simulink model "fixed_model"  (R2024a)
settings: Solver=VariableStepAuto  StartTime=0.0  StopTime=2  RelTol=1e-3
undefined symbols (not defined in the file or in its folder): Radix, SAMPLING_FREQ, signal_1
libraries: dspstat3 x3, dspsrcs4 x1, dspxfrm3 x1, simulink x1
settings Model: SimulationMode=accelerator  Creator=Jan Rosa  LastModifiedBy=Jan Rosa
settings DebuggingCC: SignalRangeChecking=warning
settings HardwareCC: ProdBitPerPointer=32  ProdBitPerSizeT=32  ProdBitPerPtrDiffT=32  ProdLargestAtomicFloat=None  ProdIntDivRoundTo=Undefined  ProdEndianess=Unspecified  ProdWordSize=32  ProdHWDeviceType=ASIC/FPGA->ASIC/FPGA  TargetBitPerPointer=64  TargetBitPerSizeT=64  TargetBitPerPtrDiffT=64  TargetLongLongMode=on  TargetIntDivRoundTo=Zero  TargetEndianess=LittleEndian  TargetWordSize=64  TargetHWDeviceType=Custom Processor->MATLAB Host Computer  ProdEqTarget=off

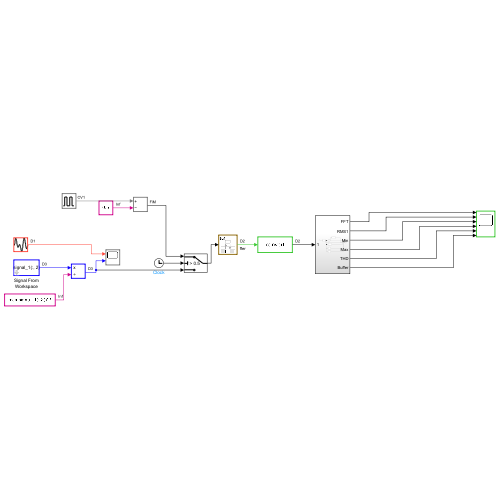
[thumbnail: Simulink's stored preview of the top-level diagram]
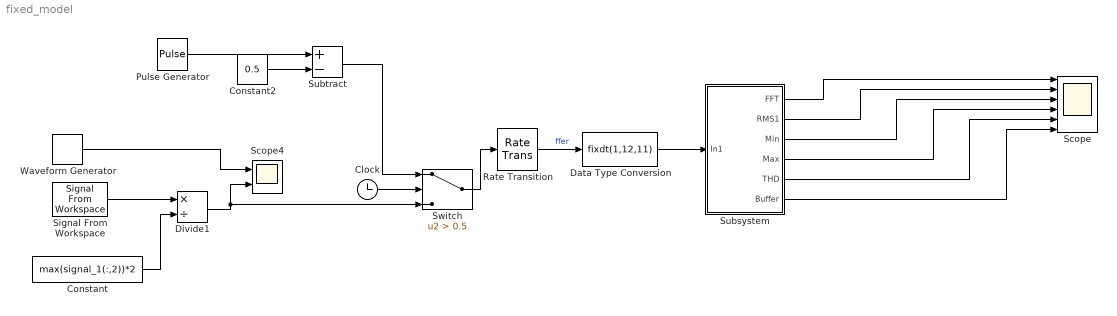
== system fixed_model ==
  Clock : Clock
  Constant : Constant  Value=max(signal_1(:,2))*2
  Constant2 : Constant  Value=0.5
  Data Type Conversion : DataTypeConversion  OutDataTypeStr=fixdt(1,12,11)  SaturateOnIntegerOverflow=off  RndMeth=Floor
  Divide1 : Product  Inputs=*/
  Pulse Generator : DiscretePulseGenerator  PulseType=Time based  Amplitude=0.999  Period=1/50  PulseWidth=50
  Rate Transition : RateTransition  Deterministic=off  OutPortSampleTime=1/SAMPLING_FREQ
  Scope : Scope  NumInputPorts=6
  Scope4 : Scope  NumInputPorts=2
  Signal From Workspace : dspsrcs4/Signal From Workspace  X=signal_1(:, 2)  Ts=signal_1(2, 1)  nsamps=1  OutputAfterFinalValue=Cyclic repetition  ignoreOrWarnInputAndFrameLengths=off  OutputFrames=off
  Subsystem : Subsystem
  Subtract : Sum  Inputs=+-
  Switch : Switch  Criteria=u2 > Threshold  Threshold=0.5  SaturateOnIntegerOverflow=off  InputSameDT=off
  Waveform Generator : simulink/Sources/Waveform Generator  OutMin=[]  OutMax=[]  OutDataTypeStr=double  SelectedSignal=1  Signals=0.99*sin(0.5, 50*2*pi, 0)  BlockNames=MultiportSwitch_c7ceefe4d1e8441  SampleTime=1/(SAMPLING_FREQ*2)
  wires:
  Rate Transition/1 -> Data Type Conversion/1  "ffer"
  Signal From Workspace/1 -> Divide1/1
  Constant/1 -> Divide1/2
  Waveform Generator/1 -> Scope4/1
  Divide1/1 -> Switch/3, Scope4/2
  Pulse Generator/1 -> Subtract/1
  Constant2/1 -> Subtract/2
  Data Type Conversion/1 -> Subsystem/1(In1)
  Subsystem/1(FFT) -> Scope/1
  Subsystem/2(RMS1) -> Scope/2
  Subsystem/3(Min) -> Scope/3
  Subsystem/4(Max) -> Scope/4
  Subsystem/5(THD) -> Scope/5
  Subsystem/6(Buffer) -> Scope/6
  Clock/1 -> Switch/2
  Subtract/1 -> Switch/1
  Switch/1 -> Rate Transition/1

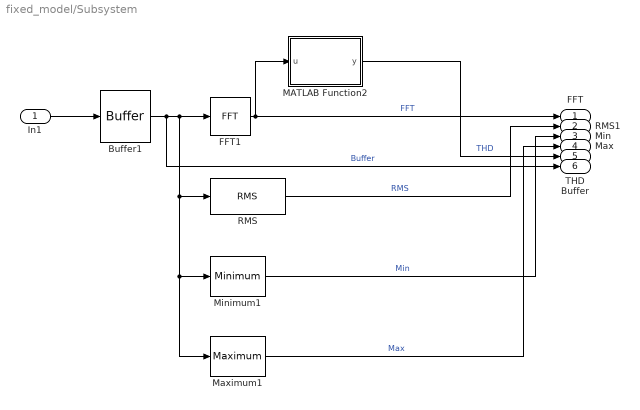
== system fixed_model/Subsystem ==
  In1 : Inport
  Buffer1 : Buffer  N=2048  V=2047  OutputFrames=off
  FFT1 : dspxfrm3/FFT  FFTImplementation=Radix-2  CompMethod=Table lookup  TableOpt=NEW  TableOptActive=Speed  BitRevOrder=off  Normalize=on  InheritFFTLength=on  FFTLength=64  WrapInput=on  roundingMode=Ceiling  overflowMode=off  firstCoeffDataTypeStr=Inherit: Same word length as input  firstCoeffLastDataTypeStr=Inherit: Same word length as input  outputMin=[]  outputMax=[]
  MATLAB Function2 : MATLAB Function  TreatAsAtomicUnit=on
  Maximum1 : dspstat3/Maximum  operation=maximum  fcn=Value  indexBase=One  operateOver=Each column  Dimension=1  InputProcessing=Columns as channels (frame based)  reset=None  roiEnable=off  roiType=Rectangles  roiPortion=Entire ROI  roiOutput=Individual statistics for each ROI  roiFlag=off  roundingMode=Floor  overflowMode=off  accumDataTypeStr=Inherit: Same as product output  accumLastDataTypeStr=Inherit: Same as product output
  Minimum1 : dspstat3/Minimum  operation=minimum  fcn=Value  indexBase=One  operateOver=Entire input  Dimension=1  InputProcessing=Columns as channels (frame based)  reset=None  roiEnable=off  roiType=Rectangles  roiPortion=Entire ROI  roiOutput=Individual statistics for each ROI  roiFlag=off  roundingMode=Floor  overflowMode=off
      settings: LibrarySourceBlock=dsphdlsupportstat/Minimum
  RMS : dspstat3/RMS  run=off  directionMode=Entire input  dimension=1  InputProcessing=Columns as channels (frame based)  reset_popup=None
  FFT : Outport
  RMS1 : Outport  Port=2
  Min : Outport  Port=3
  Max : Outport  Port=4
  THD : Outport  Port=5
  Buffer : Outport  Port=6
  wires:
  RMS/1 -> RMS1/1  "RMS"
  Maximum1/1 -> Max/1  "Max"
  Buffer1/1 -> Buffer/1, FFT1/1, Maximum1/1, Minimum1/1, RMS/1  "Buffer"
  FFT1/1 -> FFT/1, MATLAB Function2/1(u)  "FFT"
  In1/1 -> Buffer1/1
  MATLAB Function2/1(y) -> THD/1  "THD"
  Minimum1/1 -> Min/1  "Min"

== matlab function fixed_model/Subsystem/MATLAB Function2 ==
  data: u input; y output
function y = myTHD(u)

    u_abs = abs(u);
    [main_frequency_abs, main_frequency_index] = max(u_abs);
    halfway_index = floor(length(u_abs) / 2); % Calculate the halfway point
    u_abs_square = u_abs(main_frequency_index+1:halfway_index).^2;
    u_abs_SM = sum(u_abs_square);
    
y = (sqrt(u_abs_SM))/main_frequency_abs;
